simulink library "Gamepad_Xbox"  (R2025a)
settings: Solver=VariableStepAuto  StartTime=0.0  StopTime=10.0  RelTol=1e-3
libraries: vrlib x1
Description:
  | Component of Simscape Vehicle Templates Library
  | 
  | Copyright 2018-2025 The MathWorks, Inc.
settings Model: Creator=jjansev  LastModifiedBy=smiller
settings SolverCC: AlgebraicLoopSolver=TrustRegion
settings DataIOCC: ReturnWorkspaceOutputs=off
settings DebuggingCC: UnconnectedInputMsg=warning  UnconnectedOutputMsg=warning  UnconnectedLineMsg=warning  ArithmeticOperatorsInVariantConditions=warning
settings ModelReferenceCC: EnableRefExpFcnMdlSchedulingChecks=on
settings SFSimCC: CustomCodeUndefinedFunction=UseInterfaceOnly
settings RTWCC: GPUComputeCapability=3.5  DLArmComputeVersion=19.05

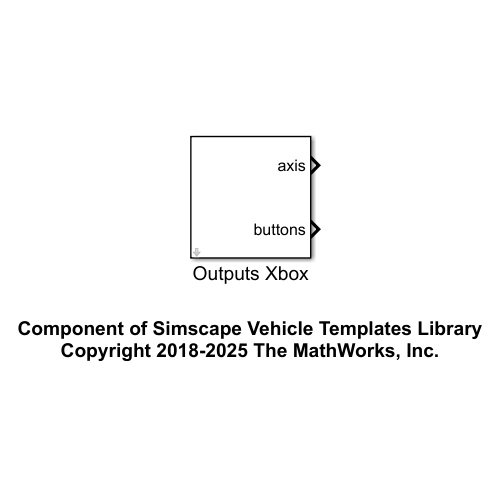
[thumbnail: Simulink's stored preview of the top-level diagram]
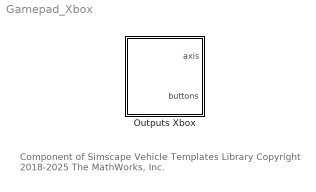
== system Gamepad_Xbox ==
  note: Component of Simscape Vehicle Templates Library
      | Copyright 2018-2025 The MathWorks, Inc.
  Outputs Xbox : Subsystem  mask{DLx=0.07, DLy=0.05, Dz=0.01, DRx=0.04, DRy=0.01, joyid=1}
      mask prompts: DLx "Left Analog stick Deadzone (Left-Right)"; DLy "Left Analog stick Deadzone (Up-Down)"; Dz "Analog Trigger Deadzone"; DRx "Right Analog stick Deadzone (Left-Right)"; DRy "Right Analog stick Deadzone (Up-Down)"; joyid "Controller ID:"
      mask init:
      | adjustports = 1;
      | forcefeed = 1;
      mask DialogControl CS_ Prompt: Dead zone setup for analog sticks
      mask DialogControl CS__copy Prompt: Controller ID Number
      mask Display: %image('D:\OneDrive - MathWorks\AE\GIT\DriverLoopVDBSSimulator\main\Libraries\Dualshock\DualShock3.png');

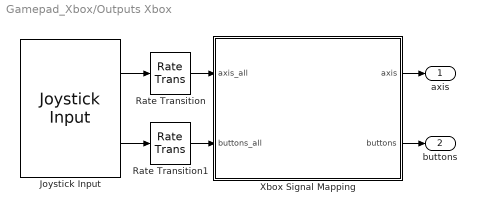
== system Gamepad_Xbox/Outputs Xbox ==
  Joystick Input : vrlib/Joystick Input  joyid=1  adjustports=on  forcefeed=off
  Rate Transition : RateTransition
  Rate Transition1 : RateTransition
  Xbox Signal Mapping : Subsystem
  axis : Outport  VectorParamsAs1DForOutWhenUnconnected=off
  buttons : Outport  Port=2  VectorParamsAs1DForOutWhenUnconnected=off
  wires:
  Xbox Signal Mapping/1(axis) -> axis/1
  Joystick Input/2 -> Rate Transition1/1
  Xbox Signal Mapping/2(buttons) -> buttons/1
  Joystick Input/1 -> Rate Transition/1
  Rate Transition/1 -> Xbox Signal Mapping/1(axis_all)
  Rate Transition1/1 -> Xbox Signal Mapping/2(buttons_all)

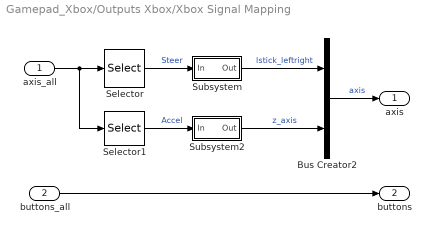
== system Gamepad_Xbox/Outputs Xbox/Xbox Signal Mapping ==
  axis_all : Inport
  buttons_all : Inport  Port=2
  Bus Creator2 : BusCreator  Inputs=2
  Selector : Selector  InputPortWidth=8  IndexOptions=Index vector (dialog)  Indices=1  OutputSizes=1
  Selector1 : Selector  InputPortWidth=8  IndexOptions=Index vector (dialog)  Indices=3  OutputSizes=1
  Subsystem : Subsystem  mask{DZ=DLx}
      mask prompts: DZ "Dead zone size (Positive numer)"
  Subsystem2 : Subsystem  mask{DZ=Dz}
      mask prompts: DZ "Dead zone size (Positive numer)"
  axis : Outport  Unit=1  VectorParamsAs1DForOutWhenUnconnected=off
  buttons : Outport  Port=2  Unit=1  VectorParamsAs1DForOutWhenUnconnected=off
  wires:
  buttons_all/1 -> buttons/1
  Bus Creator2/1 -> axis/1  "axis"
  axis_all/1 -> Selector/1, Selector1/1
  Selector/1 -> Subsystem/1(In)  "Steer"
  Selector1/1 -> Subsystem2/1(In)  "Accel"
  Subsystem/1(Out) -> Bus Creator2/1  "lstick_leftright"
  Subsystem2/1(Out) -> Bus Creator2/2  "z_axis"

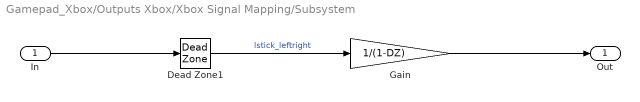
== system Gamepad_Xbox/Outputs Xbox/Xbox Signal Mapping/Subsystem ==
  In : Inport
  Dead Zone1 : DeadZone  LowerValue=-DZ  UpperValue=DZ
  Gain : Gain  Gain=1/(1-DZ)
  Out : Outport  VectorParamsAs1DForOutWhenUnconnected=off
  wires:
  Gain/1 -> Out/1
  Dead Zone1/1 -> Gain/1  "lstick_leftright"
  In/1 -> Dead Zone1/1

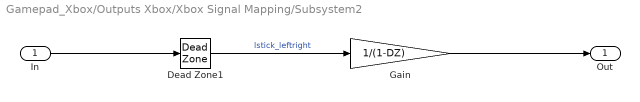
== system Gamepad_Xbox/Outputs Xbox/Xbox Signal Mapping/Subsystem2 ==
  In : Inport
  Dead Zone1 : DeadZone  LowerValue=-DZ  UpperValue=DZ
  Gain : Gain  Gain=1/(1-DZ)
  Out : Outport  VectorParamsAs1DForOutWhenUnconnected=off
  wires:
  Gain/1 -> Out/1
  Dead Zone1/1 -> Gain/1  "lstick_leftright"
  In/1 -> Dead Zone1/1
